simulink model "Attitude_Determination_Gyro"  (R2016b)
settings: Solver=FixedStepDiscrete  StartTime=0.0  StopTime=1  FixedStep=0.1  RelTol=1e-3
undefined symbols (not defined in the file or in its folder): km, s
libraries: dspmathops x4, aerolibtransform2 x1, aerolibgravity2 x1, aerolibcelestial x1
settings Model: Creator=Patipan  LastModifiedBy=Patipan

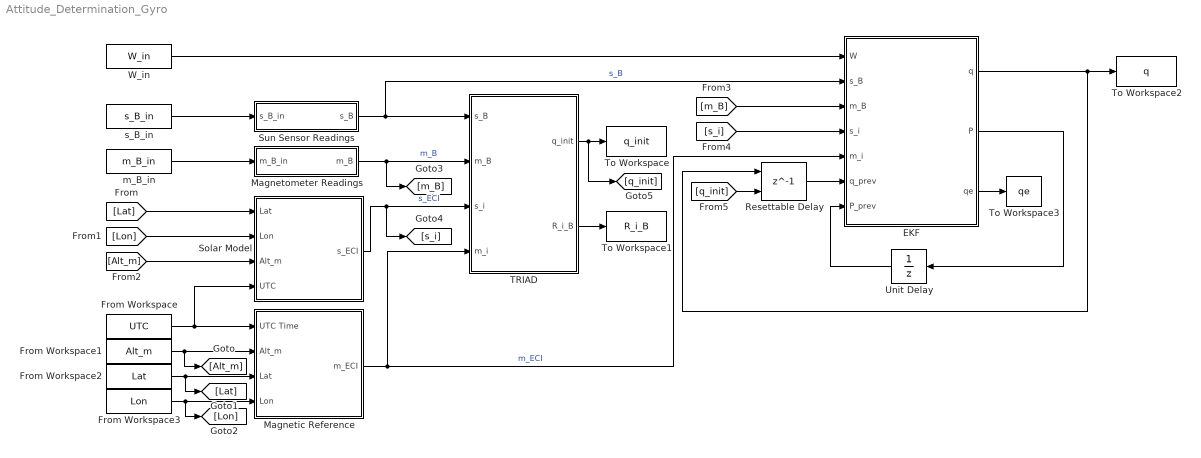
== system Attitude_Determination_Gyro ==
  EKF : MATLAB Function  TreatAsAtomicUnit=on
  From Workspace : FromWorkspace  VariableName=UTC  SampleTime=0
  From Workspace1 : FromWorkspace  VariableName=Alt_m  SampleTime=0
  From Workspace2 : FromWorkspace  VariableName=Lat  SampleTime=0
  From Workspace3 : FromWorkspace  VariableName=Lon  SampleTime=0
  Magnetic Reference : Subsystem
  Magnetometer Readings : Subsystem
  Resettable Delay : Delay  DelayLength=1  InitialConditionSource=Input port  InputProcessing=Inherited
      settings: InputPortMap=u0,p4
  Solar Model : Subsystem
  Sun Sensor Readings : Subsystem
  TRIAD : MATLAB Function  TreatAsAtomicUnit=on
  To Workspace : ToWorkspace  VariableName=q_init  SampleTime=-1
      settings: Save2DSignal=2-D array (concatenate along first dimension)
  To Workspace1 : ToWorkspace  VariableName=R_i_B  SampleTime=-1
  To Workspace2 : ToWorkspace  VariableName=q  SampleTime=-1
      settings: Save2DSignal=2-D array (concatenate along first dimension)
  To Workspace3 : ToWorkspace  VariableName=qe  SampleTime=-1
      settings: Save2DSignal=2-D array (concatenate along first dimension)
  Unit Delay : UnitDelay  InitialCondition="[1 0 0; 0  1 0; 0 0 1]"  SampleTime=-1
  W_in : FromWorkspace  VariableName=W_in  SampleTime=0
  m_B_in : FromWorkspace  VariableName=m_B_in  SampleTime=0
  "s_B_in " : FromWorkspace  VariableName=s_B_in  SampleTime=0
  wires:
  Sun Sensor Readings/1(s_B) -> EKF/2(s_B), TRIAD/1(s_B)  "s_B"
  Magnetometer Readings/1(m_B) -> [m_B], TRIAD/2(m_B)  "m_B"
  Solar Model/1(s_ECI) -> [s_i], TRIAD/3(s_i)  "s_ECI"
  Magnetic Reference/1(m_ECI) -> EKF/5(m_i), TRIAD/4(m_i)  "m_ECI"
  TRIAD/1(q_init) -> [q_init], To Workspace/1
  TRIAD/2(R_i_B) -> To Workspace1/1
  "s_B_in "/1 -> Sun Sensor Readings/1(s_B_in)
  m_B_in/1 -> Magnetometer Readings/1(m_B_in)
  From Workspace/1 -> Solar Model/4(UTC), Magnetic Reference/1(UTC Time)
  From Workspace1/1 -> [Alt_m], Magnetic Reference/2(Alt_m)
  From Workspace2/1 -> [Lat], Magnetic Reference/3(Lat)
  From Workspace3/1 -> [Lon], Magnetic Reference/4(Lon)
  [Lat] -> Solar Model/1(Lat)
  [Lon] -> Solar Model/2(Lon)
  [Alt_m] -> Solar Model/3(Alt_m)
  W_in/1 -> EKF/1(W)
  EKF/2(P) -> Unit Delay/1
  Unit Delay/1 -> EKF/7(P_prev)
  EKF/1(q) -> To Workspace2/1, Resettable Delay/1
  [s_i] -> EKF/4(s_i)
  [m_B] -> EKF/3(m_B)
  [q_init] -> Resettable Delay/2
  Resettable Delay/1 -> EKF/6(q_prev)
  EKF/3(qe) -> To Workspace3/1

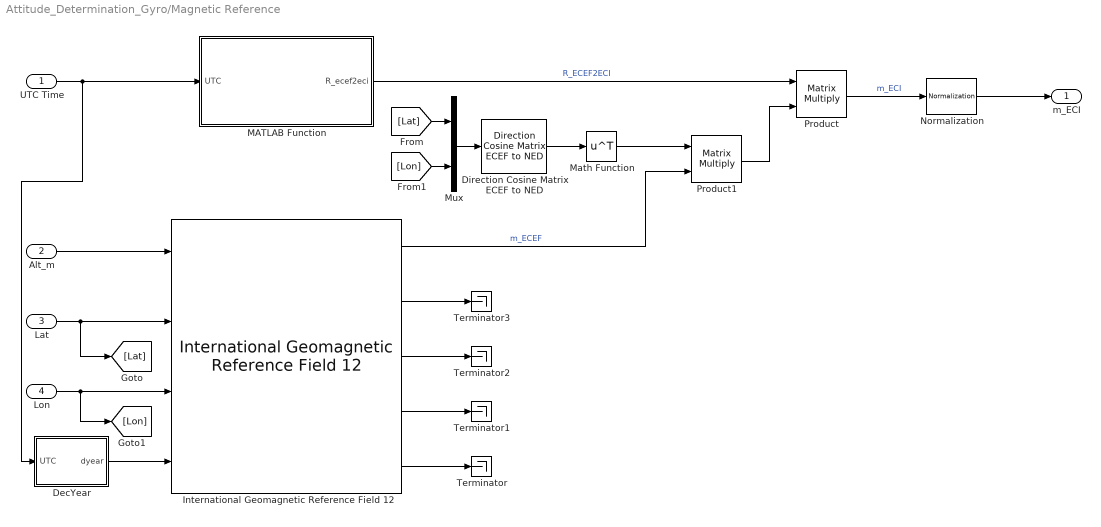
== system Attitude_Determination_Gyro/Magnetic Reference ==
  UTC Time : Inport
  Alt_m : Inport  Port=2
  Lat : Inport  Port=3
  Lon : Inport  Port=4
  DecYear : MATLAB Function  TreatAsAtomicUnit=on
  Direction Cosine Matrix ECEF to NED : aerolibtransform2/Direction Cosine Matrix ECEF to NED
  International Geomagnetic Reference Field 12 : aerolibgravity2/International Geomagnetic Reference Field 12  units=Metric (MKS)  time_in=on  month=January  day=1  year=2020  action=None  sv_out=off
  MATLAB Function : MATLAB Function  TreatAsAtomicUnit=on
  Math Function : Math  Operator=transpose  SaturateOnIntegerOverflow=on
  Mux : Mux  Inputs=2
  Normalization : dspmathops/Normalization  NormType=2-norm  Bias=1e-10  NormOver=Each column  Dimension=1  outputDataTypeStr=Inherit: Same as product output  outputLastDataTypeStr=Inherit: Same as product output  outputMin=[]  outputMax=[]  accumDataTypeStr=Inherit: Same as product output  accumLastDataTypeStr=Inherit: Same as product output  roundingMode=Floor  overflowMode=off
  Product : Product  Multiplication=Matrix(*)
  Product1 : Product  Multiplication=Matrix(*)
  Terminator{,1..3} (4 alike) : Terminator
  m_ECI : Outport
  wires:
  International Geomagnetic Reference Field 12/2 -> Terminator3/1
  International Geomagnetic Reference Field 12/3 -> Terminator2/1
  MATLAB Function/1(R_ecef2eci) -> Product/1  "R_ECEF2ECI"
  Product/1 -> Normalization/1  "m_ECI"
  International Geomagnetic Reference Field 12/4 -> Terminator1/1
  International Geomagnetic Reference Field 12/5 -> Terminator/1
  Lon/1 -> [Lon], International Geomagnetic Reference Field 12/3
  UTC Time/1 -> DecYear/1(UTC), MATLAB Function/1(UTC)
  Alt_m/1 -> International Geomagnetic Reference Field 12/1
  Lat/1 -> [Lat], International Geomagnetic Reference Field 12/2
  DecYear/1(dyear) -> International Geomagnetic Reference Field 12/4
  Mux/1 -> Direction Cosine Matrix ECEF to NED/1
  [Lat] -> Mux/1
  [Lon] -> Mux/2
  International Geomagnetic Reference Field 12/1 -> Product1/2  "m_ECEF"
  Direction Cosine Matrix ECEF to NED/1 -> Math Function/1
  Math Function/1 -> Product1/1
  Product1/1 -> Product/2
  Normalization/1 -> m_ECI/1

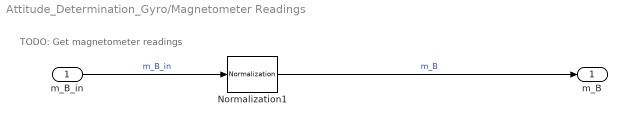
== system Attitude_Determination_Gyro/Magnetometer Readings ==
  note: TODO: Get magnetometer readings
  m_B_in : Inport
  Normalization1 : dspmathops/Normalization  NormType=2-norm  Bias=1e-10  NormOver=Each column  Dimension=1  outputDataTypeStr=Inherit: Same as product output  outputLastDataTypeStr=Inherit: Same as product output  outputMin=[]  outputMax=[]  accumDataTypeStr=Inherit: Same as product output  accumLastDataTypeStr=Inherit: Same as product output  roundingMode=Floor  overflowMode=off
  m_B : Outport
  wires:
  Normalization1/1 -> m_B/1  "m_B"
  m_B_in/1 -> Normalization1/1  "m_B_in"

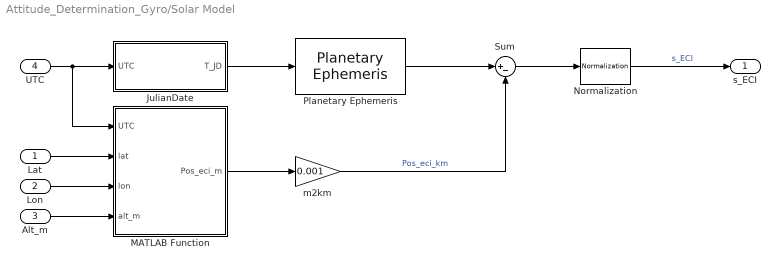
== system Attitude_Determination_Gyro/Solar Model ==
  Lat : Inport
  Lon : Inport  Port=2
  Alt_m : Inport  Port=3
  UTC : Inport  Port=4
  JulianDate : MATLAB Function  TreatAsAtomicUnit=on
  MATLAB Function : MATLAB Function  TreatAsAtomicUnit=on
  Normalization : dspmathops/Normalization  NormType=2-norm  Bias=1e-10  NormOver=Each column  Dimension=1  outputDataTypeStr=Inherit: Same as product output  outputLastDataTypeStr=Inherit: Same as product output  outputMin=[]  outputMax=[]  accumDataTypeStr=Inherit: Same as product output  accumLastDataTypeStr=Inherit: Same as product output  roundingMode=Floor  overflowMode=off
  Planetary Ephemeris : aerolibcelestial/Planetary Ephemeris  kmflag=km,km/s  epochflag=Julian date  de=DE423  nCenter=Earth  nTarget=Sun  errorflag=Error  velflag=off
  Sum : Sum  Inputs=|+-
  m2km : Gain  Gain=0.001
  s_ECI : Outport
  wires:
  Normalization/1 -> s_ECI/1  "s_ECI"
  JulianDate/1(T_JD) -> Planetary Ephemeris/1
  UTC/1 -> MATLAB Function/1(UTC), JulianDate/1(UTC)
  Lat/1 -> MATLAB Function/2(lat)
  Lon/1 -> MATLAB Function/3(lon)
  Alt_m/1 -> MATLAB Function/4(alt_m)
  MATLAB Function/1(Pos_eci_m) -> m2km/1
  Planetary Ephemeris/1 -> Sum/1
  m2km/1 -> Sum/2  "Pos_eci_km"
  Sum/1 -> Normalization/1

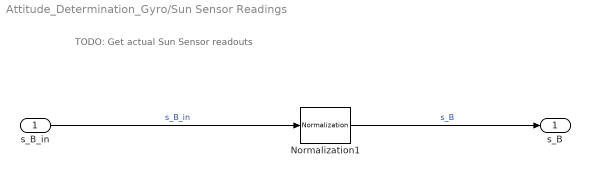
== system Attitude_Determination_Gyro/Sun Sensor Readings ==
  note: TODO: Get actual Sun Sensor readouts
  s_B_in : Inport
  Normalization1 : dspmathops/Normalization  NormType=2-norm  Bias=1e-10  NormOver=Each column  Dimension=1  outputDataTypeStr=Inherit: Same as product output  outputLastDataTypeStr=Inherit: Same as product output  outputMin=[]  outputMax=[]  accumDataTypeStr=Inherit: Same as product output  accumLastDataTypeStr=Inherit: Same as product output  roundingMode=Floor  overflowMode=off
  s_B : Outport
  wires:
  Normalization1/1 -> s_B/1  "s_B"
  s_B_in/1 -> Normalization1/1  "s_B_in"

== matlab function Attitude_Determination_Gyro/Magnetic Reference/MATLAB Function ==
  data: UTC input; R_ecef2eci output
function R_ecef2eci  = ecef2eci(UTC)
% Output rotation matrix from Earth-Centered Earth-Fixed frame to Earth
% Inertial frame from UTC time array.
%  

coder.extrinsic('dcmeci2ecef')

R_eci2ecef = zeros(3, 3);
R_eci2ecef = dcmeci2ecef('IAU-76/FK5', UTC');

R_ecef2eci = R_eci2ecef';
end

== matlab function Attitude_Determination_Gyro/TRIAD ==
  data: s_B input; m_B input; q_init output; s_i input; m_i input; R_i_B output
function [q_init, R_i_B] = TRIAD(s_B, m_B, s_i, m_i)
% This function computes attitude quaternion and rotation matrix from
% intertial to body coordinate frame using the TRIAD algorithm. See
% reference: http://www.dept.aoe.vt.edu/~cdhall/courses/aoe4140/attde.pdf
%
% This solution is only used to initialize the attitude for the EKF
%
% INPUT:
% s_B       Sun vector in body frame from sun sensors
% m_B       Magnetic field vector in body frame from magnetometers
% s_i       Sun vector in inertial frame from planetary ephemeris model
% m_i       Magnetic field vector in inertial frame from IGRF model
%
% OUTPUT:  
% q         Attitude quaternion of the satellite
% R_i_B     Rotation matrix from inertial to body
%
% Patipan Pipatpinyopong
% 11/5/16
% Modified:
%
%%%%%%%%%%%%%%%%%%%%%%%%%%%%%%%%%%%%%%%%%%%%%%%%%%%%%%%%%%%%%%%%%%%%%%%%%%%

% Assume magnetometer is more accurate. If not, will have to swap order of
% cross products

% Compute second base vector
t2b = cross(m_B, s_B)/norm(cross(m_B, s_B));
t2i = cross(m_i, s_i)/norm(cross(m_i, s_i));

% Compute third base vector to complete triad
t3b = cross(m_B, t2b);
t3i = cross(m_i, t2i);

% Construct 2 rotation matrices
A = [m_B   t2b   t3b];
B = [m_i   t2i   t3i];

% Compute rotation matrix
R_i_B = A*B';

% Convert to quaternion
% Declare extrinsic function
coder.extrinsic('dcm2quat');
q_init = [0 0 0 0];
q_init = dcm2quat(R_i_B); % q(1) is scalar
% Make sure positive scalar value
if q_init(1) < 0 
    q_init = -q_init;
end

== matlab function Attitude_Determination_Gyro/Solar Model/JulianDate ==
  data: UTC input; T_JD output
function T_JD = JulianDate(UTC)

coder.extrinsic('juliandate')
T_JD = 0;
T_JD = juliandate(UTC');

== matlab function Attitude_Determination_Gyro/Magnetic Reference/DecYear ==
  data: UTC input; dyear output
function dyear = DecYear(UTC)

coder.extrinsic('decyear');
dyear = 0;
dyear = decyear(UTC');

== matlab function Attitude_Determination_Gyro/Solar Model/MATLAB Function ==
  data: UTC input; Pos_eci_m output; lat input; lon input; alt_m input
function Pos_eci_m  = lla2eci(UTC, lat, lon, alt_m)
% Output rotation matrix from Earth-Centered Earth-Fixed frame to Earth
% Inertial frame from UTC time array.
%  

coder.extrinsic('lla2eci')

Pos_eci_m = zeros(3, 1);
Pos_eci_m = lla2eci([lat lon alt_m], UTC');

end

== matlab function Attitude_Determination_Gyro/EKF ==
  data: W input; s_B input; m_B input; s_i input; m_i input; q output; q_prev input; P_prev input; P output; qe output
function [q, P, qe] = EKF(W, s_B, m_B, s_i, m_i, q_prev, P_prev)
% This function is the extended kalman filter for CubeSat attitude
% determination.
% INPUT:
% s_B       Sun vector in body frame from sun sensors
% m_B       Magnetic field vector in body frame from magnetometers
% s_i       Sun vector in inertial frame from planetary ephemeris model
% m_i       Magnetic field vector in inertial frame from IGRF model
% q_prev    Previous attitude quaternion estimate
% P_prev    Previous state error covariance
%
% OUTPUT:  
% q         Attitude quaternion estimate of the satellite
% P         State errir covariance
%

dt = 0.1; % period for data processing
%% CubeSat ADCS - Gyro integration
% W = [wx wy wz] = [W(1) W(2) W(3)] % rotational velocity
% qdot = 0.5*B*q  quaternion derivative
% q = [q0 q_vector]'  quaternion convention used
B = [0    -W(1)   -W(2)  -W(3);
     W(1)  0      W(3)   -W(2);
     W(2)  -W(3)  0      W(1);
     W(3)  W(2)   -W(1)  0];
dq = 0.5.*(B*q_prev)'; % [1x4] vector
qgyro = q_prev' + dt.*dq; % [1x4] vector
q = quatnormalize(qgyro); % [1x4] vector
if q(1) < 0
    q = -q;
end
P = eye(3);
qe = [1 0 0 0];
